simulink model "lab_2_of_simulink"  (R2021a)
settings: Solver=VariableStepAuto  StartTime=0.0  StopTime=10.0  MaxStep=1e-3  RelTol=1e-3
settings Model: Creator=YasserNet  LastModifiedBy=YasserNet

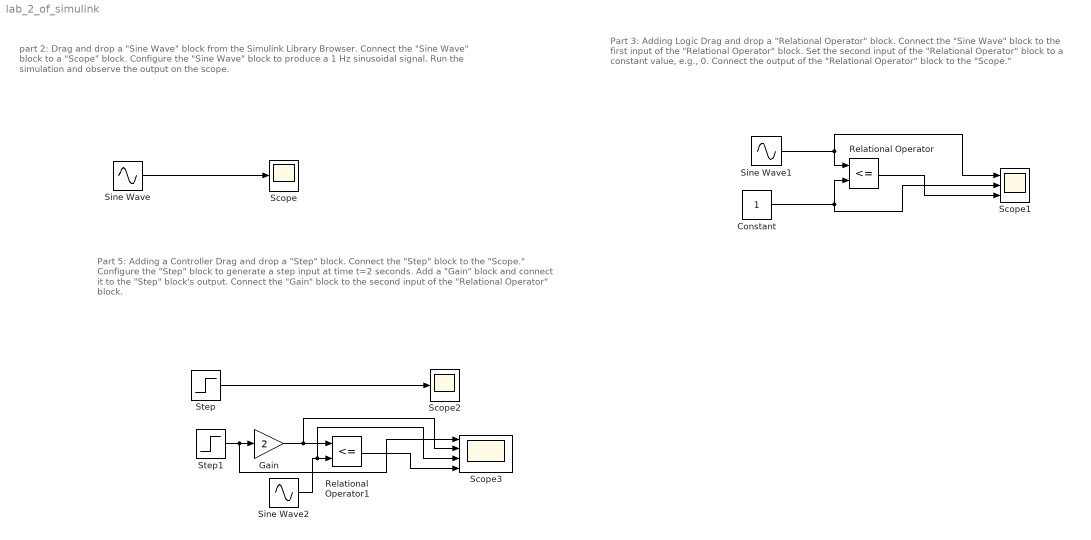
== system lab_2_of_simulink ==
  note: Part 5: Adding a Controller
      |
      | Drag and drop a "Step" block.
      | Connect the "Step" block to the "Scope."
      | Configure the "Step" block to generate a step input at time t=2 seconds.
      | Add a "Gain" block and connect it to the "Step" block's output.
      | Connect the "Gain" block to the second input of the "Relational Operator" block.
  note: Part 3: Adding Logic
      |
      | Drag and drop a "Relational Operator" block.
      | Connect the "Sine Wave" block to the first input of the "Relational Operator" block.
      | Set the second input of the "Relational Operator" block to a constant value, e.g., 0.
      | Connect the output of the "Relational Operator" block to the "Scope."
  note: part 2:
      | Drag and drop a "Sine Wave" block from the Simulink Library Browser.
      | Connect the "Sine Wave" block to a "Scope" block.
      | Configure the "Sine Wave" block to produce a 1 Hz sinusoidal signal.
      | Run the simulation and observe the output on the scope.
  Constant : Constant
  Gain : Gain  Gain=2
  Relational Operator : RelationalOperator  Operator=<=  OutDataTypeStr=boolean  RndMeth=Simplest
  Relational Operator1 : RelationalOperator  Operator=<=  OutDataTypeStr=boolean  RndMeth=Simplest
  Scope : Scope
  Scope1 : Scope  NumInputPorts=3
  Scope2 : Scope
  Scope3 : Scope  NumInputPorts=4
  Sine Wave : Sin  Amplitude=5  Frequency=2*pi  SampleTime=0
  Sine Wave1 : Sin  Amplitude=5  Frequency=2*pi  SampleTime=0
  Sine Wave2 : Sin  Frequency=2*pi  SampleTime=0
  Step : Step  Time=2  SampleTime=0
  Step1 : Step  Time=2  SampleTime=0
  wires:
  Sine Wave/1 -> Scope/1
  Relational Operator/1 -> Scope1/3
  Sine Wave1/1 -> Relational Operator/1, Scope1/1
  Constant/1 -> Relational Operator/2, Scope1/2
  Step/1 -> Scope2/1
  Gain/1 -> Scope3/2, Relational Operator1/1
  Sine Wave2/1 -> Scope3/3, Relational Operator1/2
  Step1/1 -> Scope3/1, Gain/1
  Relational Operator1/1 -> Scope3/4
